simulink model "CryoDetHcd"  (R2016b)
settings: Solver=ode45  StartTime=0.0  StopTime=1e-3  RelTol=1e-3
PreLoadFcn:
  | setup_hcd
values from neighbouring files (symbols this model uses):
  A = sqrt(0.5*erfc(x))    [setup_hcd.m]
  etaRomData = zeros(1,128)    [setup_hcd.m]
  Fadc = 614e6    (= 614000000)    [setup_hcd.m]
  freqRomData = zeros(1,128)    [setup_hcd.m]
  freqRomData1 = zeros(1,128)    [setup_hcd.m]
  freqRomData2 = zeros(1,128)    [setup_hcd.m]
  freqRomData3 = zeros(1,128)    [setup_hcd.m]
undefined symbols (not defined in the file or in its folder): AXI4, B, C, D, j, Lite
libraries: xbsIndex_r4 x2151, CryoDetLibCMB x28, hdlsllib x8, dspsigops x2, simulink x1
(part 9 of 17)

== system CryoDetHcd/DspCore/DSP/channel_processor/channel_processor_x4/freqWord_debug/alpha_filter ==
  In1 : Inport
  alpha : Inport  Port=2
  ch : Inport  Port=3
  (D-A)*B + C : xbsIndex_r4/DSP48 Macro 3.0   dsptype=Target XtremeDSP Slice: DSP48E2  instruction_list=(D-A)*B+C  AvailableInstructions=|  show_filtered=on  pipeline_options=Expert  dspimage=?  tier_1=off  tier_2=off  tier_3=off  tier_4=off  tier_5=off  tier_6=off  dreg_1=off  dreg_2=off  dreg_3=on  areg_1=off  areg_2=off  areg_3=on  areg_4=on  breg_1=off  breg_2=off  breg_3=on  breg_4=on  mreg_5=on  concatreg_3=off  concatreg_4=off  concatreg_5=off  creg_1=off  creg_2=off  creg_3=on  creg_4=on  creg_5=on  preg_6=on  cinreg_1=off  cinreg_2=off  cinreg_3=off  cinreg_4=off  cinreg_5=off  opreg_1=off  opreg_2=off  opreg_3=off  opreg_4=off  opreg_5=off  output_properties=Full_Precision  p_width=48  p_binarywidth=0  has_acout=off  has_bcout=off  has_pcout=off  has_carryout=off  has_carrycascout=off  has_ce=off  has_d_ce=off  has_a_ce=off  has_b_ce=off  has_concat_ce=off  has_c_ce=off  has_m_ce=off  has_p_ce=off  has_sel_ce=off  has_sclr=off  has_d_sclr=off  has_a_sclr=off  has_b_sclr=off  has_concat_sclr=off  has_c_sclr=off  has_m_sclr=off  has_p_sclr=off  has_sel_sclr=off  use_dsp48=on  simulation_type=fast_sim  simulation_model=sysgen:xbip_dsp48_macro_v3_0  gui_behaviour=Sysgen  instruction1='#'  ip_name=DSP48 Macro  ip_version=3.0  dsptool_ready=true  ipcore_usecache=true  ipcore_useipmodelcache=true  wrapper_available=true  port_translation_map={ 'ce' => 'en', 'sclr' => 'rst'}  ipcore_latency_function='has_combinational'  structural_sim=false  ipcore_verbose=false  ipcore_port_config={ 'carryin' => { 'arith' => 'ufix', 'binpt' => 0.00000000000, 'width' => 1.00000000000}, 'carrycascin' => { 'arith' => 'ufix', 'binpt' => 0.00000000000, 'width' => 1.00000000000}, 'carrycascout' => { 'arith' => 'ufix', 'binpt' => 0.00000000000, 'width' => 1.00000000000}, 'carryout' => { 'arith' => 'ufix', 'binpt' => 0.00000000000, 'width' => 1.00000000000}}  ipcore_xco_need_fpga_part=true  block_type=xbip_dsp48_macro_v3_0
      | (D-A)*B+C
      | (D-A)*B+C+C
      | (D-A)*B+C+C+CARRYIN
      | (D-A)*B+C+CARRYIN
      | (D-A)*B+C+P
      | (D-A)*B+C+P+CARRYIN
      | (D-A)*B+C+P>>17
      | (D-A)*B+C+P>>17+CARRYIN
      | (D-A)*B+C+PCIN
      | (D-A)*B+C+PCIN+CARRYIN
      | (D-A)*B+C+PCIN>>17
      | (D-A)*B+C+PCIN>>17+CARRYIN
      | (D-A)*B+C-C
      | (D-A)*B+C-P
      | (D-A)*B+C-P>>17
      | (D-A)*B+C-PCIN
      | (D-A)*B+C-PCIN>>17
      | (D-A)*B+CARRYIN
      | -((D-A)*B+C)
      | -((D-A)*B+C+CARRYIN)
      | -((D-A)*B+CARRYIN)
      | -(C+(D-A)*B+CARRYIN)
      | -(P+(D-A)*B+CARRYIN)
      | -C+(D-A)*B+C
      | -P+(D-A)*B+C
      | -P>>17+(D-A)*B+C
      | -PCIN+(D-A)*B+C
      | -PCIN>>17+(D-A)*B+C
      | C+(D-A)*B+C
      | C+(D-A)*B+C+CARRYIN
      | C+(D-A)*B+CARRYIN
      | C+C+(D-A)*B+CARRYIN
      | C+P+(D-A)*B+CARRYIN
      | C+P>>17+(D-A)*B+CARRYIN
      | C+PCIN+(D-A)*B+CARRYIN
      | C+PCIN>>17+(D-A)*B+CARRYIN
      | C-((D-A)*B+C)
      | C-((D-A)*B+C+CARRYIN)
      | C-((D-A)*B+CARRYIN)
      | C-(C+(D-A)*B+CARRYIN)
      | C-(P+(D-A)*B+CARRYIN)
      | P+(D-A)*B+C
      | P+(D-A)*B+C+CARRYIN
      | P+(D-A)*B+CARRYIN
      | P+C+(D-A)*B+CARRYIN
      | P+P+(D-A)*B+CARRYIN
      | P+P>>17+(D-A)*B+CARRYIN
      | P+PCIN+(D-A)*B+CARRYIN
      | P+PCIN>>17+(D-A)*B+CARRYIN
      | P-((D-A)*B+C)
      | P-((D-A)*B+C+CARRYIN)
      | P-((D-A)*B+CARRYIN)
      | P-(C+(D-A)*B+CARRYIN)
      | P-(P+(D-A)*B+CARRYIN)
      | P>>17+(D-A)*B+C
      | P>>17+(D-A)*B+C+CARRYIN
      | P>>17+(D-A)*B+CARRYIN
      | P>>17+C+(D-A)*B+CARRYIN
      | P>>17+P+(D-A)*B+CARRYIN
      | P>>17-((D-A)*B+C)
      | P>>17-((D-A)*B+C+CARRYIN)
      | P>>17-((D-A)*B+CARRYIN)
      | P>>17-(C+(D-A)*B+CARRYIN)
      | P>>17-(P+(D-A)*B+CARRYIN)
      | PCIN+(D-A)*B+C
      | PCIN+(D-A)*B+C+CARRYIN
      | PCIN+(D-A)*B+CARRYIN
      | PCIN+C+(D-A)*B+CARRYIN
      | PCIN+P+(D-A)*B+CARRYIN
      | PCIN-((D-A)*B+C)
      | PCIN-((D-A)*B+C+CARRYIN)
      | PCIN-((D-A)*B+CARRYIN)
      | PCIN-(C+(D-A)*B+CARRYIN)
      | PCIN-(P+(D-A)*B+CARRYIN)
      | PCIN>>17+(D-A)*B+C
      | PCIN>>17+(D-A)*B+C+CARRYIN
      | PCIN>>17+(D-A)*B+CARRYIN
      | PCIN>>17+C+(D-A)*B+CARRYIN
      | PCIN>>17+P+(D-A)*B+CARRYIN
      | PCIN>>17-((D-A)*B+C)
      | PCIN>>17-((D-A)*B+C+CARRYIN)
      | PCIN>>17-((D-A)*B+CARRYIN)
      | PCIN>>17-(C+(D-A)*B+CARRYIN)
      | PCIN>>17-(P+(D-A)*B+CARRYIN)
      | RNDMACC((D-A)*B+C+P)
      | RNDSIMPLE((D-A)*B+C)
      | RNDSIMPLE((D-A)*B+C+CARRYIN)
      | RNDSIMPLE((D-A)*B+CARRYIN)
      | RNDSIMPLE(C+(D-A)*B+CARRYIN)
      | RNDSIMPLE(P+(D-A)*B+CARRYIN)
      | RNDSIMPLE(P>>17+(D-A)*B+CARRYIN)
      | RNDSIMPLE(PCIN+(D-A)*B+CARRYIN)
      | RNDSIMPLE(PCIN>>17+(D-A)*B+CARRYIN)
      settings: infoedit=<html>Valid operands: CONCAT, P, C, PCIN, P>>17, PCIN>>17, CARRYIN, CARRYCASCIN, ACIN, A, BCIN,B<br><br>Valid operators: +, -, *, ()<br><br>Valid functions: RNDSIMPLE, RNDSYM<br><br>Instructions are case insensitive and tolerate spaces.</html>
  Convert : xbsIndex_r4/Convert  gui_display_data_type=Fixed-point  arith_type=Unsigned  n_bits=24  bin_pt=0  float_type=Single  exp_bits=8  fraction_bits=24  quantization=Truncate  overflow=Wrap  en=off  latency=0  pipeline=off  dbl_ovrd=off  block_type=convert
  Convert1 : xbsIndex_r4/Convert  gui_display_data_type=Fixed-point  arith_type="Signed  (2's comp)"  n_bits=25  bin_pt=0  float_type=Single  exp_bits=8  fraction_bits=24  quantization=Truncate  overflow=Wrap  en=off  latency=0  pipeline=off  dbl_ovrd=off  block_type=convert
  Convert2 : xbsIndex_r4/Convert  gui_display_data_type=Fixed-point  arith_type="Signed  (2's comp)"  n_bits=18  bin_pt=15  float_type=Single  exp_bits=8  fraction_bits=24  quantization=Truncate  overflow=Wrap  en=off  latency=0  pipeline=off  dbl_ovrd=off  block_type=convert
  Convert3 : xbsIndex_r4/Convert  gui_display_data_type=Fixed-point  arith_type="Signed  (2's comp)"  n_bits=25  bin_pt=0  float_type=Single  exp_bits=8  fraction_bits=24  quantization=Truncate  overflow=Wrap  en=off  latency=0  pipeline=off  dbl_ovrd=off  block_type=convert
  Delay : xbsIndex_r4/Delay  rst=off  infoeditControl=Selection of Reset will increase slice count due to use of real FFs and instead of SRLs  en=off  latency=4  reg_retiming=off  dbl_ovrd=off  block_type=delay
  Delay1 : xbsIndex_r4/Delay  rst=off  infoeditControl=Selection of Reset will increase slice count due to use of real FFs and instead of SRLs  en=off  latency=4  reg_retiming=off  dbl_ovrd=off  block_type=delay
  Register : xbsIndex_r4/Register  init=0  rst=off  en=off  dbl_ovrd=off  block_type=register
  Out1 : Outport
  ch_o : Outport  Port=2
  wires:
  Register/1 -> Convert3/1
  In1/1 -> Register/1
  Delay/1 -> Convert1/1, (D-A)*B + C/4
  (D-A)*B + C/1 -> Convert/1, Delay/1
  Convert1/1 -> (D-A)*B + C/2
  Convert/1 -> Out1/1
  Convert2/1 -> (D-A)*B + C/3
  Convert3/1 -> (D-A)*B + C/1
  ch/1 -> Delay1/1
  Delay1/1 -> ch_o/1
  alpha/1 -> Convert2/1

== system CryoDetHcd/DspCore/DSP/channel_processor/channel_processor_x4/freqWord_debug/alpha_filter1 ==
  In1 : Inport
  alpha : Inport  Port=2
  ch : Inport  Port=3
  (D-A)*B + C : xbsIndex_r4/DSP48 Macro 3.0   dsptype=Target XtremeDSP Slice: DSP48E2  instruction_list=(D-A)*B+C  AvailableInstructions=|  show_filtered=on  pipeline_options=Expert  dspimage=?  tier_1=off  tier_2=off  tier_3=off  tier_4=off  tier_5=off  tier_6=off  dreg_1=off  dreg_2=off  dreg_3=on  areg_1=off  areg_2=off  areg_3=on  areg_4=on  breg_1=off  breg_2=off  breg_3=on  breg_4=on  mreg_5=on  concatreg_3=off  concatreg_4=off  concatreg_5=off  creg_1=off  creg_2=off  creg_3=on  creg_4=on  creg_5=on  preg_6=on  cinreg_1=off  cinreg_2=off  cinreg_3=off  cinreg_4=off  cinreg_5=off  opreg_1=off  opreg_2=off  opreg_3=off  opreg_4=off  opreg_5=off  output_properties=Full_Precision  p_width=48  p_binarywidth=0  has_acout=off  has_bcout=off  has_pcout=off  has_carryout=off  has_carrycascout=off  has_ce=off  has_d_ce=off  has_a_ce=off  has_b_ce=off  has_concat_ce=off  has_c_ce=off  has_m_ce=off  has_p_ce=off  has_sel_ce=off  has_sclr=off  has_d_sclr=off  has_a_sclr=off  has_b_sclr=off  has_concat_sclr=off  has_c_sclr=off  has_m_sclr=off  has_p_sclr=off  has_sel_sclr=off  use_dsp48=on  simulation_type=fast_sim  simulation_model=sysgen:xbip_dsp48_macro_v3_0  gui_behaviour=Sysgen  instruction1='#'  ip_name=DSP48 Macro  ip_version=3.0  dsptool_ready=true  ipcore_usecache=true  ipcore_useipmodelcache=true  wrapper_available=true  port_translation_map={ 'ce' => 'en', 'sclr' => 'rst'}  ipcore_latency_function='has_combinational'  structural_sim=false  ipcore_verbose=false  ipcore_port_config={ 'carryin' => { 'arith' => 'ufix', 'binpt' => 0.00000000000, 'width' => 1.00000000000}, 'carrycascin' => { 'arith' => 'ufix', 'binpt' => 0.00000000000, 'width' => 1.00000000000}, 'carrycascout' => { 'arith' => 'ufix', 'binpt' => 0.00000000000, 'width' => 1.00000000000}, 'carryout' => { 'arith' => 'ufix', 'binpt' => 0.00000000000, 'width' => 1.00000000000}}  ipcore_xco_need_fpga_part=true  block_type=xbip_dsp48_macro_v3_0
      | (D-A)*B+C
      | (D-A)*B+C+C
      | (D-A)*B+C+C+CARRYIN
      | (D-A)*B+C+CARRYIN
      | (D-A)*B+C+P
      | (D-A)*B+C+P+CARRYIN
      | (D-A)*B+C+P>>17
      | (D-A)*B+C+P>>17+CARRYIN
      | (D-A)*B+C+PCIN
      | (D-A)*B+C+PCIN+CARRYIN
      | (D-A)*B+C+PCIN>>17
      | (D-A)*B+C+PCIN>>17+CARRYIN
      | (D-A)*B+C-C
      | (D-A)*B+C-P
      | (D-A)*B+C-P>>17
      | (D-A)*B+C-PCIN
      | (D-A)*B+C-PCIN>>17
      | (D-A)*B+CARRYIN
      | -((D-A)*B+C)
      | -((D-A)*B+C+CARRYIN)
      | -((D-A)*B+CARRYIN)
      | -(C+(D-A)*B+CARRYIN)
      | -(P+(D-A)*B+CARRYIN)
      | -C+(D-A)*B+C
      | -P+(D-A)*B+C
      | -P>>17+(D-A)*B+C
      | -PCIN+(D-A)*B+C
      | -PCIN>>17+(D-A)*B+C
      | C+(D-A)*B+C
      | C+(D-A)*B+C+CARRYIN
      | C+(D-A)*B+CARRYIN
      | C+C+(D-A)*B+CARRYIN
      | C+P+(D-A)*B+CARRYIN
      | C+P>>17+(D-A)*B+CARRYIN
      | C+PCIN+(D-A)*B+CARRYIN
      | C+PCIN>>17+(D-A)*B+CARRYIN
      | C-((D-A)*B+C)
      | C-((D-A)*B+C+CARRYIN)
      | C-((D-A)*B+CARRYIN)
      | C-(C+(D-A)*B+CARRYIN)
      | C-(P+(D-A)*B+CARRYIN)
      | P+(D-A)*B+C
      | P+(D-A)*B+C+CARRYIN
      | P+(D-A)*B+CARRYIN
      | P+C+(D-A)*B+CARRYIN
      | P+P+(D-A)*B+CARRYIN
      | P+P>>17+(D-A)*B+CARRYIN
      | P+PCIN+(D-A)*B+CARRYIN
      | P+PCIN>>17+(D-A)*B+CARRYIN
      | P-((D-A)*B+C)
      | P-((D-A)*B+C+CARRYIN)
      | P-((D-A)*B+CARRYIN)
      | P-(C+(D-A)*B+CARRYIN)
      | P-(P+(D-A)*B+CARRYIN)
      | P>>17+(D-A)*B+C
      | P>>17+(D-A)*B+C+CARRYIN
      | P>>17+(D-A)*B+CARRYIN
      | P>>17+C+(D-A)*B+CARRYIN
      | P>>17+P+(D-A)*B+CARRYIN
      | P>>17-((D-A)*B+C)
      | P>>17-((D-A)*B+C+CARRYIN)
      | P>>17-((D-A)*B+CARRYIN)
      | P>>17-(C+(D-A)*B+CARRYIN)
      | P>>17-(P+(D-A)*B+CARRYIN)
      | PCIN+(D-A)*B+C
      | PCIN+(D-A)*B+C+CARRYIN
      | PCIN+(D-A)*B+CARRYIN
      | PCIN+C+(D-A)*B+CARRYIN
      | PCIN+P+(D-A)*B+CARRYIN
      | PCIN-((D-A)*B+C)
      | PCIN-((D-A)*B+C+CARRYIN)
      | PCIN-((D-A)*B+CARRYIN)
      | PCIN-(C+(D-A)*B+CARRYIN)
      | PCIN-(P+(D-A)*B+CARRYIN)
      | PCIN>>17+(D-A)*B+C
      | PCIN>>17+(D-A)*B+C+CARRYIN
      | PCIN>>17+(D-A)*B+CARRYIN
      | PCIN>>17+C+(D-A)*B+CARRYIN
      | PCIN>>17+P+(D-A)*B+CARRYIN
      | PCIN>>17-((D-A)*B+C)
      | PCIN>>17-((D-A)*B+C+CARRYIN)
      | PCIN>>17-((D-A)*B+CARRYIN)
      | PCIN>>17-(C+(D-A)*B+CARRYIN)
      | PCIN>>17-(P+(D-A)*B+CARRYIN)
      | RNDMACC((D-A)*B+C+P)
      | RNDSIMPLE((D-A)*B+C)
      | RNDSIMPLE((D-A)*B+C+CARRYIN)
      | RNDSIMPLE((D-A)*B+CARRYIN)
      | RNDSIMPLE(C+(D-A)*B+CARRYIN)
      | RNDSIMPLE(P+(D-A)*B+CARRYIN)
      | RNDSIMPLE(P>>17+(D-A)*B+CARRYIN)
      | RNDSIMPLE(PCIN+(D-A)*B+CARRYIN)
      | RNDSIMPLE(PCIN>>17+(D-A)*B+CARRYIN)
      settings: infoedit=<html>Valid operands: CONCAT, P, C, PCIN, P>>17, PCIN>>17, CARRYIN, CARRYCASCIN, ACIN, A, BCIN,B<br><br>Valid operators: +, -, *, ()<br><br>Valid functions: RNDSIMPLE, RNDSYM<br><br>Instructions are case insensitive and tolerate spaces.</html>
  Convert : xbsIndex_r4/Convert  gui_display_data_type=Fixed-point  arith_type=Unsigned  n_bits=24  bin_pt=0  float_type=Single  exp_bits=8  fraction_bits=24  quantization=Truncate  overflow=Wrap  en=off  latency=0  pipeline=off  dbl_ovrd=off  block_type=convert
  Convert1 : xbsIndex_r4/Convert  gui_display_data_type=Fixed-point  arith_type="Signed  (2's comp)"  n_bits=25  bin_pt=0  float_type=Single  exp_bits=8  fraction_bits=24  quantization=Truncate  overflow=Wrap  en=off  latency=0  pipeline=off  dbl_ovrd=off  block_type=convert
  Convert2 : xbsIndex_r4/Convert  gui_display_data_type=Fixed-point  arith_type="Signed  (2's comp)"  n_bits=18  bin_pt=15  float_type=Single  exp_bits=8  fraction_bits=24  quantization=Truncate  overflow=Wrap  en=off  latency=0  pipeline=off  dbl_ovrd=off  block_type=convert
  Convert3 : xbsIndex_r4/Convert  gui_display_data_type=Fixed-point  arith_type="Signed  (2's comp)"  n_bits=25  bin_pt=0  float_type=Single  exp_bits=8  fraction_bits=24  quantization=Truncate  overflow=Wrap  en=off  latency=0  pipeline=off  dbl_ovrd=off  block_type=convert
  Delay : xbsIndex_r4/Delay  rst=off  infoeditControl=Selection of Reset will increase slice count due to use of real FFs and instead of SRLs  en=off  latency=4  reg_retiming=off  dbl_ovrd=off  block_type=delay
  Delay1 : xbsIndex_r4/Delay  rst=off  infoeditControl=Selection of Reset will increase slice count due to use of real FFs and instead of SRLs  en=off  latency=4  reg_retiming=off  dbl_ovrd=off  block_type=delay
  Register : xbsIndex_r4/Register  init=0  rst=off  en=off  dbl_ovrd=off  block_type=register
  Out1 : Outport
  ch_o : Outport  Port=2
  wires:
  alpha/1 -> Convert2/1
  Delay1/1 -> ch_o/1
  ch/1 -> Delay1/1
  Convert3/1 -> (D-A)*B + C/1
  Convert2/1 -> (D-A)*B + C/3
  Convert/1 -> Out1/1
  Convert1/1 -> (D-A)*B + C/2
  (D-A)*B + C/1 -> Delay/1, Convert/1
  Delay/1 -> (D-A)*B + C/4, Convert1/1
  In1/1 -> Register/1
  Register/1 -> Convert3/1

== system CryoDetHcd/DspCore/DSP/channel_processor/channel_processor_x4/freqWord_debug/alpha_filter2 ==
  In1 : Inport
  alpha : Inport  Port=2
  ch : Inport  Port=3
  (D-A)*B + C : xbsIndex_r4/DSP48 Macro 3.0   dsptype=Target XtremeDSP Slice: DSP48E2  instruction_list=(D-A)*B+C  AvailableInstructions=|  show_filtered=on  pipeline_options=Expert  dspimage=?  tier_1=off  tier_2=off  tier_3=off  tier_4=off  tier_5=off  tier_6=off  dreg_1=off  dreg_2=off  dreg_3=on  areg_1=off  areg_2=off  areg_3=on  areg_4=on  breg_1=off  breg_2=off  breg_3=on  breg_4=on  mreg_5=on  concatreg_3=off  concatreg_4=off  concatreg_5=off  creg_1=off  creg_2=off  creg_3=on  creg_4=on  creg_5=on  preg_6=on  cinreg_1=off  cinreg_2=off  cinreg_3=off  cinreg_4=off  cinreg_5=off  opreg_1=off  opreg_2=off  opreg_3=off  opreg_4=off  opreg_5=off  output_properties=Full_Precision  p_width=48  p_binarywidth=0  has_acout=off  has_bcout=off  has_pcout=off  has_carryout=off  has_carrycascout=off  has_ce=off  has_d_ce=off  has_a_ce=off  has_b_ce=off  has_concat_ce=off  has_c_ce=off  has_m_ce=off  has_p_ce=off  has_sel_ce=off  has_sclr=off  has_d_sclr=off  has_a_sclr=off  has_b_sclr=off  has_concat_sclr=off  has_c_sclr=off  has_m_sclr=off  has_p_sclr=off  has_sel_sclr=off  use_dsp48=on  simulation_type=fast_sim  simulation_model=sysgen:xbip_dsp48_macro_v3_0  gui_behaviour=Sysgen  instruction1='#'  ip_name=DSP48 Macro  ip_version=3.0  dsptool_ready=true  ipcore_usecache=true  ipcore_useipmodelcache=true  wrapper_available=true  port_translation_map={ 'ce' => 'en', 'sclr' => 'rst'}  ipcore_latency_function='has_combinational'  structural_sim=false  ipcore_verbose=false  ipcore_port_config={ 'carryin' => { 'arith' => 'ufix', 'binpt' => 0.00000000000, 'width' => 1.00000000000}, 'carrycascin' => { 'arith' => 'ufix', 'binpt' => 0.00000000000, 'width' => 1.00000000000}, 'carrycascout' => { 'arith' => 'ufix', 'binpt' => 0.00000000000, 'width' => 1.00000000000}, 'carryout' => { 'arith' => 'ufix', 'binpt' => 0.00000000000, 'width' => 1.00000000000}}  ipcore_xco_need_fpga_part=true  block_type=xbip_dsp48_macro_v3_0
      | (D-A)*B+C
      | (D-A)*B+C+C
      | (D-A)*B+C+C+CARRYIN
      | (D-A)*B+C+CARRYIN
      | (D-A)*B+C+P
      | (D-A)*B+C+P+CARRYIN
      | (D-A)*B+C+P>>17
      | (D-A)*B+C+P>>17+CARRYIN
      | (D-A)*B+C+PCIN
      | (D-A)*B+C+PCIN+CARRYIN
      | (D-A)*B+C+PCIN>>17
      | (D-A)*B+C+PCIN>>17+CARRYIN
      | (D-A)*B+C-C
      | (D-A)*B+C-P
      | (D-A)*B+C-P>>17
      | (D-A)*B+C-PCIN
      | (D-A)*B+C-PCIN>>17
      | (D-A)*B+CARRYIN
      | -((D-A)*B+C)
      | -((D-A)*B+C+CARRYIN)
      | -((D-A)*B+CARRYIN)
      | -(C+(D-A)*B+CARRYIN)
      | -(P+(D-A)*B+CARRYIN)
      | -C+(D-A)*B+C
      | -P+(D-A)*B+C
      | -P>>17+(D-A)*B+C
      | -PCIN+(D-A)*B+C
      | -PCIN>>17+(D-A)*B+C
      | C+(D-A)*B+C
      | C+(D-A)*B+C+CARRYIN
      | C+(D-A)*B+CARRYIN
      | C+C+(D-A)*B+CARRYIN
      | C+P+(D-A)*B+CARRYIN
      | C+P>>17+(D-A)*B+CARRYIN
      | C+PCIN+(D-A)*B+CARRYIN
      | C+PCIN>>17+(D-A)*B+CARRYIN
      | C-((D-A)*B+C)
      | C-((D-A)*B+C+CARRYIN)
      | C-((D-A)*B+CARRYIN)
      | C-(C+(D-A)*B+CARRYIN)
      | C-(P+(D-A)*B+CARRYIN)
      | P+(D-A)*B+C
      | P+(D-A)*B+C+CARRYIN
      | P+(D-A)*B+CARRYIN
      | P+C+(D-A)*B+CARRYIN
      | P+P+(D-A)*B+CARRYIN
      | P+P>>17+(D-A)*B+CARRYIN
      | P+PCIN+(D-A)*B+CARRYIN
      | P+PCIN>>17+(D-A)*B+CARRYIN
      | P-((D-A)*B+C)
      | P-((D-A)*B+C+CARRYIN)
      | P-((D-A)*B+CARRYIN)
      | P-(C+(D-A)*B+CARRYIN)
      | P-(P+(D-A)*B+CARRYIN)
      | P>>17+(D-A)*B+C
      | P>>17+(D-A)*B+C+CARRYIN
      | P>>17+(D-A)*B+CARRYIN
      | P>>17+C+(D-A)*B+CARRYIN
      | P>>17+P+(D-A)*B+CARRYIN
      | P>>17-((D-A)*B+C)
      | P>>17-((D-A)*B+C+CARRYIN)
      | P>>17-((D-A)*B+CARRYIN)
      | P>>17-(C+(D-A)*B+CARRYIN)
      | P>>17-(P+(D-A)*B+CARRYIN)
      | PCIN+(D-A)*B+C
      | PCIN+(D-A)*B+C+CARRYIN
      | PCIN+(D-A)*B+CARRYIN
      | PCIN+C+(D-A)*B+CARRYIN
      | PCIN+P+(D-A)*B+CARRYIN
      | PCIN-((D-A)*B+C)
      | PCIN-((D-A)*B+C+CARRYIN)
      | PCIN-((D-A)*B+CARRYIN)
      | PCIN-(C+(D-A)*B+CARRYIN)
      | PCIN-(P+(D-A)*B+CARRYIN)
      | PCIN>>17+(D-A)*B+C
      | PCIN>>17+(D-A)*B+C+CARRYIN
      | PCIN>>17+(D-A)*B+CARRYIN
      | PCIN>>17+C+(D-A)*B+CARRYIN
      | PCIN>>17+P+(D-A)*B+CARRYIN
      | PCIN>>17-((D-A)*B+C)
      | PCIN>>17-((D-A)*B+C+CARRYIN)
      | PCIN>>17-((D-A)*B+CARRYIN)
      | PCIN>>17-(C+(D-A)*B+CARRYIN)
      | PCIN>>17-(P+(D-A)*B+CARRYIN)
      | RNDMACC((D-A)*B+C+P)
      | RNDSIMPLE((D-A)*B+C)
      | RNDSIMPLE((D-A)*B+C+CARRYIN)
      | RNDSIMPLE((D-A)*B+CARRYIN)
      | RNDSIMPLE(C+(D-A)*B+CARRYIN)
      | RNDSIMPLE(P+(D-A)*B+CARRYIN)
      | RNDSIMPLE(P>>17+(D-A)*B+CARRYIN)
      | RNDSIMPLE(PCIN+(D-A)*B+CARRYIN)
      | RNDSIMPLE(PCIN>>17+(D-A)*B+CARRYIN)
      settings: infoedit=<html>Valid operands: CONCAT, P, C, PCIN, P>>17, PCIN>>17, CARRYIN, CARRYCASCIN, ACIN, A, BCIN,B<br><br>Valid operators: +, -, *, ()<br><br>Valid functions: RNDSIMPLE, RNDSYM<br><br>Instructions are case insensitive and tolerate spaces.</html>
  Convert : xbsIndex_r4/Convert  gui_display_data_type=Fixed-point  arith_type=Unsigned  n_bits=24  bin_pt=0  float_type=Single  exp_bits=8  fraction_bits=24  quantization=Truncate  overflow=Wrap  en=off  latency=0  pipeline=off  dbl_ovrd=off  block_type=convert
  Convert1 : xbsIndex_r4/Convert  gui_display_data_type=Fixed-point  arith_type="Signed  (2's comp)"  n_bits=25  bin_pt=0  float_type=Single  exp_bits=8  fraction_bits=24  quantization=Truncate  overflow=Wrap  en=off  latency=0  pipeline=off  dbl_ovrd=off  block_type=convert
  Convert2 : xbsIndex_r4/Convert  gui_display_data_type=Fixed-point  arith_type="Signed  (2's comp)"  n_bits=18  bin_pt=15  float_type=Single  exp_bits=8  fraction_bits=24  quantization=Truncate  overflow=Wrap  en=off  latency=0  pipeline=off  dbl_ovrd=off  block_type=convert
  Convert3 : xbsIndex_r4/Convert  gui_display_data_type=Fixed-point  arith_type="Signed  (2's comp)"  n_bits=25  bin_pt=0  float_type=Single  exp_bits=8  fraction_bits=24  quantization=Truncate  overflow=Wrap  en=off  latency=0  pipeline=off  dbl_ovrd=off  block_type=convert
  Delay : xbsIndex_r4/Delay  rst=off  infoeditControl=Selection of Reset will increase slice count due to use of real FFs and instead of SRLs  en=off  latency=4  reg_retiming=off  dbl_ovrd=off  block_type=delay
  Delay1 : xbsIndex_r4/Delay  rst=off  infoeditControl=Selection of Reset will increase slice count due to use of real FFs and instead of SRLs  en=off  latency=4  reg_retiming=off  dbl_ovrd=off  block_type=delay
  Register : xbsIndex_r4/Register  init=0  rst=off  en=off  dbl_ovrd=off  block_type=register
  Out1 : Outport
  ch_o : Outport  Port=2
  wires:
  Register/1 -> Convert3/1
  In1/1 -> Register/1
  Delay/1 -> Convert1/1, (D-A)*B + C/4
  (D-A)*B + C/1 -> Convert/1, Delay/1
  Convert1/1 -> (D-A)*B + C/2
  Convert/1 -> Out1/1
  Convert2/1 -> (D-A)*B + C/3
  Convert3/1 -> (D-A)*B + C/1
  ch/1 -> Delay1/1
  Delay1/1 -> ch_o/1
  alpha/1 -> Convert2/1

== system CryoDetHcd/DspCore/DSP/channel_processor/channel_processor_x4/freqWord_debug/alpha_filter3 ==
  In1 : Inport
  alpha : Inport  Port=2
  ch : Inport  Port=3
  (D-A)*B + C : xbsIndex_r4/DSP48 Macro 3.0   dsptype=Target XtremeDSP Slice: DSP48E2  instruction_list=(D-A)*B+C  AvailableInstructions=|  show_filtered=on  pipeline_options=Expert  dspimage=?  tier_1=off  tier_2=off  tier_3=off  tier_4=off  tier_5=off  tier_6=off  dreg_1=off  dreg_2=off  dreg_3=on  areg_1=off  areg_2=off  areg_3=on  areg_4=on  breg_1=off  breg_2=off  breg_3=on  breg_4=on  mreg_5=on  concatreg_3=off  concatreg_4=off  concatreg_5=off  creg_1=off  creg_2=off  creg_3=on  creg_4=on  creg_5=on  preg_6=on  cinreg_1=off  cinreg_2=off  cinreg_3=off  cinreg_4=off  cinreg_5=off  opreg_1=off  opreg_2=off  opreg_3=off  opreg_4=off  opreg_5=off  output_properties=Full_Precision  p_width=48  p_binarywidth=0  has_acout=off  has_bcout=off  has_pcout=off  has_carryout=off  has_carrycascout=off  has_ce=off  has_d_ce=off  has_a_ce=off  has_b_ce=off  has_concat_ce=off  has_c_ce=off  has_m_ce=off  has_p_ce=off  has_sel_ce=off  has_sclr=off  has_d_sclr=off  has_a_sclr=off  has_b_sclr=off  has_concat_sclr=off  has_c_sclr=off  has_m_sclr=off  has_p_sclr=off  has_sel_sclr=off  use_dsp48=on  simulation_type=fast_sim  simulation_model=sysgen:xbip_dsp48_macro_v3_0  gui_behaviour=Sysgen  instruction1='#'  ip_name=DSP48 Macro  ip_version=3.0  dsptool_ready=true  ipcore_usecache=true  ipcore_useipmodelcache=true  wrapper_available=true  port_translation_map={ 'ce' => 'en', 'sclr' => 'rst'}  ipcore_latency_function='has_combinational'  structural_sim=false  ipcore_verbose=false  ipcore_port_config={ 'carryin' => { 'arith' => 'ufix', 'binpt' => 0.00000000000, 'width' => 1.00000000000}, 'carrycascin' => { 'arith' => 'ufix', 'binpt' => 0.00000000000, 'width' => 1.00000000000}, 'carrycascout' => { 'arith' => 'ufix', 'binpt' => 0.00000000000, 'width' => 1.00000000000}, 'carryout' => { 'arith' => 'ufix', 'binpt' => 0.00000000000, 'width' => 1.00000000000}}  ipcore_xco_need_fpga_part=true  block_type=xbip_dsp48_macro_v3_0
      | (D-A)*B+C
      | (D-A)*B+C+C
      | (D-A)*B+C+C+CARRYIN
      | (D-A)*B+C+CARRYIN
      | (D-A)*B+C+P
      | (D-A)*B+C+P+CARRYIN
      | (D-A)*B+C+P>>17
      | (D-A)*B+C+P>>17+CARRYIN
      | (D-A)*B+C+PCIN
      | (D-A)*B+C+PCIN+CARRYIN
      | (D-A)*B+C+PCIN>>17
      | (D-A)*B+C+PCIN>>17+CARRYIN
      | (D-A)*B+C-C
      | (D-A)*B+C-P
      | (D-A)*B+C-P>>17
      | (D-A)*B+C-PCIN
      | (D-A)*B+C-PCIN>>17
      | (D-A)*B+CARRYIN
      | -((D-A)*B+C)
      | -((D-A)*B+C+CARRYIN)
      | -((D-A)*B+CARRYIN)
      | -(C+(D-A)*B+CARRYIN)
      | -(P+(D-A)*B+CARRYIN)
      | -C+(D-A)*B+C
      | -P+(D-A)*B+C
      | -P>>17+(D-A)*B+C
      | -PCIN+(D-A)*B+C
      | -PCIN>>17+(D-A)*B+C
      | C+(D-A)*B+C
      | C+(D-A)*B+C+CARRYIN
      | C+(D-A)*B+CARRYIN
      | C+C+(D-A)*B+CARRYIN
      | C+P+(D-A)*B+CARRYIN
      | C+P>>17+(D-A)*B+CARRYIN
      | C+PCIN+(D-A)*B+CARRYIN
      | C+PCIN>>17+(D-A)*B+CARRYIN
      | C-((D-A)*B+C)
      | C-((D-A)*B+C+CARRYIN)
      | C-((D-A)*B+CARRYIN)
      | C-(C+(D-A)*B+CARRYIN)
      | C-(P+(D-A)*B+CARRYIN)
      | P+(D-A)*B+C
      | P+(D-A)*B+C+CARRYIN
      | P+(D-A)*B+CARRYIN
      | P+C+(D-A)*B+CARRYIN
      | P+P+(D-A)*B+CARRYIN
      | P+P>>17+(D-A)*B+CARRYIN
      | P+PCIN+(D-A)*B+CARRYIN
      | P+PCIN>>17+(D-A)*B+CARRYIN
      | P-((D-A)*B+C)
      | P-((D-A)*B+C+CARRYIN)
      | P-((D-A)*B+CARRYIN)
      | P-(C+(D-A)*B+CARRYIN)
      | P-(P+(D-A)*B+CARRYIN)
      | P>>17+(D-A)*B+C
      | P>>17+(D-A)*B+C+CARRYIN
      | P>>17+(D-A)*B+CARRYIN
      | P>>17+C+(D-A)*B+CARRYIN
      | P>>17+P+(D-A)*B+CARRYIN
      | P>>17-((D-A)*B+C)
      | P>>17-((D-A)*B+C+CARRYIN)
      | P>>17-((D-A)*B+CARRYIN)
      | P>>17-(C+(D-A)*B+CARRYIN)
      | P>>17-(P+(D-A)*B+CARRYIN)
      | PCIN+(D-A)*B+C
      | PCIN+(D-A)*B+C+CARRYIN
      | PCIN+(D-A)*B+CARRYIN
      | PCIN+C+(D-A)*B+CARRYIN
      | PCIN+P+(D-A)*B+CARRYIN
      | PCIN-((D-A)*B+C)
      | PCIN-((D-A)*B+C+CARRYIN)
      | PCIN-((D-A)*B+CARRYIN)
      | PCIN-(C+(D-A)*B+CARRYIN)
      | PCIN-(P+(D-A)*B+CARRYIN)
      | PCIN>>17+(D-A)*B+C
      | PCIN>>17+(D-A)*B+C+CARRYIN
      | PCIN>>17+(D-A)*B+CARRYIN
      | PCIN>>17+C+(D-A)*B+CARRYIN
      | PCIN>>17+P+(D-A)*B+CARRYIN
      | PCIN>>17-((D-A)*B+C)
      | PCIN>>17-((D-A)*B+C+CARRYIN)
      | PCIN>>17-((D-A)*B+CARRYIN)
      | PCIN>>17-(C+(D-A)*B+CARRYIN)
      | PCIN>>17-(P+(D-A)*B+CARRYIN)
      | RNDMACC((D-A)*B+C+P)
      | RNDSIMPLE((D-A)*B+C)
      | RNDSIMPLE((D-A)*B+C+CARRYIN)
      | RNDSIMPLE((D-A)*B+CARRYIN)
      | RNDSIMPLE(C+(D-A)*B+CARRYIN)
      | RNDSIMPLE(P+(D-A)*B+CARRYIN)
      | RNDSIMPLE(P>>17+(D-A)*B+CARRYIN)
      | RNDSIMPLE(PCIN+(D-A)*B+CARRYIN)
      | RNDSIMPLE(PCIN>>17+(D-A)*B+CARRYIN)
      settings: infoedit=<html>Valid operands: CONCAT, P, C, PCIN, P>>17, PCIN>>17, CARRYIN, CARRYCASCIN, ACIN, A, BCIN,B<br><br>Valid operators: +, -, *, ()<br><br>Valid functions: RNDSIMPLE, RNDSYM<br><br>Instructions are case insensitive and tolerate spaces.</html>
  Convert : xbsIndex_r4/Convert  gui_display_data_type=Fixed-point  arith_type=Unsigned  n_bits=24  bin_pt=0  float_type=Single  exp_bits=8  fraction_bits=24  quantization=Truncate  overflow=Wrap  en=off  latency=0  pipeline=off  dbl_ovrd=off  block_type=convert
  Convert1 : xbsIndex_r4/Convert  gui_display_data_type=Fixed-point  arith_type="Signed  (2's comp)"  n_bits=25  bin_pt=0  float_type=Single  exp_bits=8  fraction_bits=24  quantization=Truncate  overflow=Wrap  en=off  latency=0  pipeline=off  dbl_ovrd=off  block_type=convert
  Convert2 : xbsIndex_r4/Convert  gui_display_data_type=Fixed-point  arith_type="Signed  (2's comp)"  n_bits=18  bin_pt=15  float_type=Single  exp_bits=8  fraction_bits=24  quantization=Truncate  overflow=Wrap  en=off  latency=0  pipeline=off  dbl_ovrd=off  block_type=convert
  Convert3 : xbsIndex_r4/Convert  gui_display_data_type=Fixed-point  arith_type="Signed  (2's comp)"  n_bits=25  bin_pt=0  float_type=Single  exp_bits=8  fraction_bits=24  quantization=Truncate  overflow=Wrap  en=off  latency=0  pipeline=off  dbl_ovrd=off  block_type=convert
  Delay : xbsIndex_r4/Delay  rst=off  infoeditControl=Selection of Reset will increase slice count due to use of real FFs and instead of SRLs  en=off  latency=4  reg_retiming=off  dbl_ovrd=off  block_type=delay
  Delay1 : xbsIndex_r4/Delay  rst=off  infoeditControl=Selection of Reset will increase slice count due to use of real FFs and instead of SRLs  en=off  latency=4  reg_retiming=off  dbl_ovrd=off  block_type=delay
  Register : xbsIndex_r4/Register  init=0  rst=off  en=off  dbl_ovrd=off  block_type=register
  Out1 : Outport
  ch_o : Outport  Port=2
  wires:
  alpha/1 -> Convert2/1
  Delay1/1 -> ch_o/1
  ch/1 -> Delay1/1
  Convert3/1 -> (D-A)*B + C/1
  Convert2/1 -> (D-A)*B + C/3
  Convert/1 -> Out1/1
  Convert1/1 -> (D-A)*B + C/2
  (D-A)*B + C/1 -> Delay/1, Convert/1
  Delay/1 -> (D-A)*B + C/4, Convert1/1
  In1/1 -> Register/1
  Register/1 -> Convert3/1

== system CryoDetHcd/DspCore/DSP/channel_processor/channel_processor_x4/128_channel_processor1/DDS Mixer taylor series corrected/DDS 8ch taylor series corrected ==
  note: Taylor series corrected - use 0.5 BRAM (18 bit storage, 2^10 points), 3DSP
  note: Phase Accumulator
      | (8 Channels)
  note: 8 Channel DDS
      | Given its channel ID, takes instantaneous frequency for this channel of each band and generates phase and I&Q
      | interleaved over 8 bands
      | Frequency RAM is updated asynchronously to operation
  note: don't worry about matching latency here, will do downstream
  valid : Inport
  rst : Inport  Port=2
  freqWord : Inport  Port=3
  index : Inport  Port=4
  ch : Inport  Port=5
  BitBasher : xbsIndex_r4/BitBasher  bitexpr=tmux = {in[6:4]}  display_expr=off  sr_1=tmux  arith_type1=Unsigned  bin_pt1=0  sr_2=subband  arith_type2=Unsigned  bin_pt2=0  sr_3=3  arith_type3=Unsigned  bin_pt3=0  sr_4=4  arith_type4=Unsigned  bin_pt4=0  dbl_ovrd=off  block_type=bitbasher
  BitBasher1 : xbsIndex_r4/BitBasher  bitexpr=|  display_expr=off  sr_1=ch  arith_type1=Unsigned  bin_pt1=0  sr_2=amp  arith_type2=Unsigned  bin_pt2=0  sr_3=3  arith_type3=Unsigned  bin_pt3=0  sr_4=4  arith_type4=Unsigned  bin_pt4=0  dbl_ovrd=off  block_type=bitbasher
      | ch = {in[6:4]}
      | amp = {in[3:0]}
  BitBasher2 : xbsIndex_r4/BitBasher  bitexpr=|  display_expr=off  sr_1=freq  arith_type1=Unsigned  bin_pt1=24  sr_2=amp  arith_type2=Unsigned  bin_pt2=0  sr_3=3  arith_type3=Unsigned  bin_pt3=0  sr_4=4  arith_type4=Unsigned  bin_pt4=0  dbl_ovrd=off  block_type=bitbasher
      | freq = {in[23:0]}
      | amp = {in[27:24]}
  BitBasher3 : xbsIndex_r4/BitBasher  bitexpr=out = {ch, amp}  display_expr=off  sr_1=out  arith_type1=Unsigned  bin_pt1=0  sr_2=amp  arith_type2=Unsigned  bin_pt2=0  sr_3=3  arith_type3=Unsigned  bin_pt3=0  sr_4=4  arith_type4=Unsigned  bin_pt4=0  dbl_ovrd=off  block_type=bitbasher
  BitBasher4 : xbsIndex_r4/BitBasher  bitexpr=|  display_expr=off  sr_1=ch  arith_type1=Unsigned  bin_pt1=0  sr_2=amp  arith_type2=Unsigned  bin_pt2=0  sr_3=3  arith_type3=Unsigned  bin_pt3=0  sr_4=4  arith_type4=Unsigned  bin_pt4=0  dbl_ovrd=off  block_type=bitbasher
      | ch = {in[6:4]}
      | amp = {in[3:0]}
  BitBasher5 : xbsIndex_r4/BitBasher  bitexpr=phase = {in[23:8]}  display_expr=off  sr_1=phase  arith_type1="Signed  (2's comp)"  bin_pt1=15  sr_2=amp  arith_type2=Unsigned  bin_pt2=0  sr_3=3  arith_type3=Unsigned  bin_pt3=0  sr_4=4  arith_type4=Unsigned  bin_pt4=0  dbl_ovrd=off  block_type=bitbasher
  Bus Creator : BusCreator  Inputs=3
  Counter : xbsIndex_r4/Counter  cnt_type=Free Running  cnt_to=Inf  operation=Up  start_count=0  cnt_by_val=1  arith_type=Unsigned  n_bits=3  bin_pt=0  load_pin=off  rst=on  en=on  explicit_period=off  period=1  use_behavioral_HDL=off  implementation=Fabric  dbl_ovrd=off  block_type=counter
  DDS Compiler 6.0 1 : xbsIndex_r4/DDS Compiler 6.0   partspresent=Phase_Generator_only  dds_clock_rate=100  channels=8  mode_of_operation=Standard  modulus=9  parameter_entry=System_Parameters  spurious_free_dynamic_range=45  frequency_resolution=0.4  noise_shaping=None  phase_width=24  output_width=3  output_selection=Sine_and_Cosine  negative_sine=off  negative_cosine=off  amplitude_mode=Full_Range  memory_type=Auto  optimization_goal=Auto  dsp48_use=Minimal  resync=off  latency_configuration=Auto  latency=1  has_phase_out=on  has_aclken=off  has_aresetn=on  explicit_period=off  period=1  data_has_tlast=Not_Required  has_tready=off  s_phase_has_tuser=User_Field  m_data_has_tuser=Not_Required  m_phase_has_tuser=User_Field  s_phase_tuser_width=7  output_form=Twos_Complement  s_config_sync_mode=On_Vector  phase_increment=Streaming  output_frequency1=0  output_frequency2=0  output_frequency3=0  output_frequency4=0  output_frequency5=0  output_frequency6=0  output_frequency7=0  output_frequency8=0  output_frequency9=0  output_frequency10=0  output_frequency11=0  output_frequency12=0  output_frequency13=0  output_frequency14=0  output_frequency15=0  output_frequency16=0  pinc1='0'  pinc2='0'  pinc3='0'  pinc4='0'  pinc5='0'  pinc6='0'  pinc7='0'  pinc8='0'  pinc9='0'  pinc10='0'  pinc11='0'  pinc12='0'  pinc13='0'  pinc14='0'  pinc15='0'  pinc16='0'  phase_offset=None  phase_offset_angles1=0  phase_offset_angles2=0  phase_offset_angles3=0  phase_offset_angles4=0  phase_offset_angles5=0  phase_offset_angles6=0  phase_offset_angles7=0  phase_offset_angles8=0  phase_offset_angles9=0  phase_offset_angles10=0  phase_offset_angles11=0  phase_offset_angles12=0  phase_offset_angles13=0  phase_offset_angles14=0  phase_offset_angles15=0  phase_offset_angles16=0  poff1='0'  poff2='0'  poff3='0'  poff4='0'  poff5='0'  poff6='0'  poff7='0'  poff8='0'  poff9='0'  poff10='0'  poff11='0'  poff12='0'  poff13='0'  poff14='0'  poff15='0'  poff16='0'  trim_axipin_name=on  simulation_type=hybrid_sim  simulation_model=sysgen:xddsv6_0_cmodel  data_path_portlist={ 's_axis_config_tdata_poff', 's_axis_config_tdata_chan0_poff', 's_axis_config_tdata_pinc', 's_axis_config_tdata_chan0_pinc', 's_axis_phase_tdata_resync', 's_axis_phase_tdata_chan0_resync', 's_axis_phase_tdata_poff', 's_axis_phase_tdata_chan0_poff', 's_axis_phase_tdata_pinc', 's_axis_phase_tdata_chan0_pinc', 's_axis_phase_tdata_phase_in', 'm_axis_data_tdata_sine', 'm_axis_data_tdata_chan0_sine', 'm_axis_data_tdata_cosine', 'm_axis_data_tdata_chan0_cosine', 'm_axis_phase_tdata_phase_out', 'm_axis_phase_tdata_chan0_phase_out'}  por_mode=false  gui_behaviour=Sysgen  ip_name=DDS Compiler  ip_version=6.0  dsptool_ready=true  wrapper_available=true  port_translation_map={ 'aclken' => 'en', 'aresetn' => 'rst' }  ipcore_usecache=true  ipcore_useipmodelcache=true  ipcore_xco_need_fpga_part=true  ipcore_verbose=false  block_type=dds_compiler_v6_0
  DDS Compiler 6.0 2 : xbsIndex_r4/DDS Compiler 6.0   partspresent=SIN_COS_LUT_only  dds_clock_rate=100  channels=1  mode_of_operation=Standard  modulus=9  parameter_entry=System_Parameters  spurious_free_dynamic_range=45  frequency_resolution=0.4  noise_shaping=Taylor_Series_Corrected  phase_width=24  output_width=18  output_selection=Sine_and_Cosine  negative_sine=off  negative_cosine=off  amplitude_mode=Full_Range  memory_type=Auto  optimization_goal=Area  dsp48_use=Minimal  resync=off  latency_configuration=Auto  latency=1  has_phase_out=off  has_aclken=off  has_aresetn=off  explicit_period=off  period=1  data_has_tlast=Not_Required  has_tready=off  s_phase_has_tuser=User_Field  m_data_has_tuser=User_Field  m_phase_has_tuser=Not_Required  s_phase_tuser_width=7  output_form=Twos_Complement  s_config_sync_mode=On_Vector  phase_increment=Streaming  output_frequency1=0  output_frequency2=0  output_frequency3=0  output_frequency4=0  output_frequency5=0  output_frequency6=0  output_frequency7=0  output_frequency8=0  output_frequency9=0  output_frequency10=0  output_frequency11=0  output_frequency12=0  output_frequency13=0  output_frequency14=0  output_frequency15=0  output_frequency16=0  pinc1='0'  pinc2='0'  pinc3='0'  pinc4='0'  pinc5='0'  pinc6='0'  pinc7='0'  pinc8='0'  pinc9='0'  pinc10='0'  pinc11='0'  pinc12='0'  pinc13='0'  pinc14='0'  pinc15='0'  pinc16='0'  phase_offset=Streaming  phase_offset_angles1=0  phase_offset_angles2=0  phase_offset_angles3=0  phase_offset_angles4=0  phase_offset_angles5=0  phase_offset_angles6=0  phase_offset_angles7=0  phase_offset_angles8=0  phase_offset_angles9=0  phase_offset_angles10=0  phase_offset_angles11=0  phase_offset_angles12=0  phase_offset_angles13=0  phase_offset_angles14=0  phase_offset_angles15=0  phase_offset_angles16=0  poff1='0'  poff2='0'  poff3='0'  poff4='0'  poff5='0'  poff6='0'  poff7='0'  poff8='0'  poff9='0'  poff10='0'  poff11='0'  poff12='0'  poff13='0'  poff14='0'  poff15='0'  poff16='0'  trim_axipin_name=on  simulation_type=hybrid_sim  simulation_model=sysgen:xddsv6_0_cmodel  data_path_portlist={ 's_axis_config_tdata_poff', 's_axis_config_tdata_chan0_poff', 's_axis_config_tdata_pinc', 's_axis_config_tdata_chan0_pinc', 's_axis_phase_tdata_resync', 's_axis_phase_tdata_chan0_resync', 's_axis_phase_tdata_poff', 's_axis_phase_tdata_chan0_poff', 's_axis_phase_tdata_pinc', 's_axis_phase_tdata_chan0_pinc', 's_axis_phase_tdata_phase_in', 'm_axis_data_tdata_sine', 'm_axis_data_tdata_chan0_sine', 'm_axis_data_tdata_cosine', 'm_axis_data_tdata_chan0_cosine', 'm_axis_phase_tdata_phase_out', 'm_axis_phase_tdata_chan0_phase_out'}  por_mode=false  gui_behaviour=Sysgen  ip_name=DDS Compiler  ip_version=6.0  dsptool_ready=true  wrapper_available=true  port_translation_map={ 'aclken' => 'en', 'aresetn' => 'rst' }  ipcore_usecache=true  ipcore_useipmodelcache=true  ipcore_xco_need_fpga_part=true  ipcore_verbose=false  block_type=dds_compiler_v6_0
  Inverter : xbsIndex_r4/Inverter  en=off  latency=1  dbl_ovrd=off  block_type=inv
  Register{,1..2,6..11} (9 alike) : xbsIndex_r4/Register  init=0  rst=off  en=off  dbl_ovrd=off  block_type=register
  Register3 : xbsIndex_r4/Register  init=0  rst=off  en=on  dbl_ovrd=off  block_type=register
  Register4 : xbsIndex_r4/Register  init=0  rst=off  en=on  dbl_ovrd=off  block_type=register
  Register5 : xbsIndex_r4/Register  init=0  rst=off  en=on  dbl_ovrd=off  block_type=register
  Terminator1 : Terminator
  Terminator2 : Terminator
  tuser : xbsIndex_r4/Constant  const=0  gui_display_data_type=Boolean  arith_type=Boolean  n_bits=1  bin_pt=0  preci_type=Single  exp_width=8  frac_width=24  explicit_period=off  period=1  equ=P=C  opselect=C  inp2=PCIN>>17  opr=+  inp1=P  carry=CIN  dbl_ovrd=off  block_type=constant
  valid1 : InportShadow
  valid_o : Outport
  Q : Outport  Port=2
  I : Outport  Port=3
  amp_o : Outport  Port=4
  ch_o : Outport  Port=5
  phaseBus : Outport  Port=6
  wires:
  Register10/1 -> BitBasher3/2
  Counter/1 -> Register11/1
  Register11/1 -> Register10/1
  rst/1 -> Inverter/1, Counter/1
  valid/1 -> Counter/2
  Register9/1 -> Register6/1
  Register8/1 -> Register1/1
  Register7/1 -> Register/1
  Inverter/1 -> DDS Compiler 6.0 1/5
  BitBasher5/1 -> Bus Creator/2  "phase"
  Bus Creator/1 -> phaseBus/1
  Register1/1 -> BitBasher2/1
  BitBasher4/1 -> ch_o/1
  Register5/1 -> BitBasher4/1  "INDX"
  BitBasher2/2 -> BitBasher3/1
  freqWord/1 -> Register8/1
  Register2/1 -> valid_o/1  "valid"
  Register3/1 -> Q/1  "Q"
  Register4/1 -> I/1  "I"
  BitBasher/1 -> Register7/1
  ch/1 -> BitBasher/1
  DDS Compiler 6.0 2/2 -> Register3/1  "Q"
  DDS Compiler 6.0 2/1 -> Register5/2, Register4/2, Register3/2, Register2/1  "valid"
  valid1/1 -> Register9/1
  DDS Compiler 6.0 2/3 -> Register4/1  "I"
  DDS Compiler 6.0 2/4 -> Register5/1  "INDX"
  BitBasher4/2 -> amp_o/1
  BitBasher1/1 -> Bus Creator/3  "ch"
  DDS Compiler 6.0 1/1 -> Bus Creator/1, DDS Compiler 6.0 2/1  "valid"
  BitBasher2/1 -> DDS Compiler 6.0 1/2
  BitBasher3/1 -> DDS Compiler 6.0 1/4
  Register6/1 -> DDS Compiler 6.0 1/1  "valid"
  DDS Compiler 6.0 1/2 -> DDS Compiler 6.0 2/2, BitBasher5/1  "phase"
  DDS Compiler 6.0 1/3 -> DDS Compiler 6.0 2/3, BitBasher1/1  "tyser"
  tuser/1 -> DDS Compiler 6.0 1/3
  DDS Compiler 6.0 1/4 -> Terminator1/1
  DDS Compiler 6.0 1/5 -> Terminator2/1

== system CryoDetHcd/DspCore/DSP/channel_processor/channel_processor_x4/128_channel_processor1/DDS Mixer taylor series corrected/mixer ==
  note: depth 16 should be enough
      |   8 here
      |   ~3-4 in DDS block
  note: match latency for phaseBus
  note: Need complex? Swap IQ
  note: can this be modulo 8?
  In1 : Inport
  In2 : Inport  Port=2
  phaseBus : Inport  Port=3
  BitBasher2 : xbsIndex_r4/BitBasher  bitexpr=out={Q, I}  display_expr=off  sr_1=out  arith_type1=Unsigned  bin_pt1=0  sr_2=2  arith_type2=Unsigned  bin_pt2=0  sr_3=3  arith_type3=Unsigned  bin_pt3=0  sr_4=4  arith_type4=Unsigned  bin_pt4=0  dbl_ovrd=off  block_type=bitbasher
  BitBasher3 : xbsIndex_r4/BitBasher  bitexpr=|  display_expr=off  sr_1=Q  arith_type1="Signed  (2's comp)"  bin_pt1=15  sr_2=I  arith_type2="Signed  (2's comp)"  bin_pt2=15  sr_3=I  arith_type3=Unsigned  bin_pt3=0  sr_4=4  arith_type4=Unsigned  bin_pt4=0  dbl_ovrd=off  block_type=bitbasher
      | Q = {in[31:16]}
      | I = {in[15:0]}
  Bus Creator : BusCreator  Inputs=3
  Bus Creator1 : BusCreator  Inputs=4
  Bus Selector1 : BusSelector  OutputSignals=valid,Q,I,ch
  Bus Selector2 : BusSelector  OutputSignals=valid,Q,I
  Bus Selector3 : BusSelector  OutputSignals=valid,phase,ch
  "Complex Multiplier 6.0 " : xbsIndex_r4/Complex Multiplier 6.0   hasatlast=off  hasatuser=on  atuserwidth=3  hasbtlast=off  hasbtuser=off  btuserwidth=1  multtype=Use_Mults  optimizegoal=Resources  flowcontrol=NonBlocking  outputwidth=19  roundmode=Truncate  hasctrltlast=off  hasctrltuser=off  ctrltuserwidth=1  outtlastbehv=Null  latencyconfig=Manual  minimumlatency=6  aclken=off  aresetn=off  trim_axipin_name=on  simulation_type=hybrid_sim  simulation_model=sysgen:cmpy_v6_0  data_path_portlist={ 's_axis_a_tdata_real', 's_axis_a_tdata_imag', 's_axis_b_tdata_real', 's_axis_b_tdata_imag', 's_axis_ctrl_tdata_rounding_bit', 'm_axis_dout_tdata_real', 'm_axis_dout_tdata_imag' }  aportwidth=63  bportwidth=63  ip_name=Complex Multiplier  ip_version=6.0  dsptool_ready=true  ipcore_usecache=true  ipcore_useipmodelcache=true  ipcore_verbose=false  ipcore_latency_parameter='minimumlatency'  wrapper_available=true  port_translation_map={ 'aclken' => 'en', 'aresetn' => 'rst'}  block_type=cmpy_v6_0
  Convert : xbsIndex_r4/Convert  gui_display_data_type=Fixed-point  arith_type="Signed  (2's comp)"  n_bits=18  bin_pt=16  float_type=Single  exp_bits=8  fraction_bits=24  quantization=Truncate  overflow=Wrap  en=off  latency=0  pipeline=off  dbl_ovrd=off  block_type=convert
  Convert1 : xbsIndex_r4/Convert  gui_display_data_type=Fixed-point  arith_type="Signed  (2's comp)"  n_bits=18  bin_pt=16  float_type=Single  exp_bits=8  fraction_bits=24  quantization=Truncate  overflow=Wrap  en=off  latency=0  pipeline=off  dbl_ovrd=off  block_type=convert
  Delay : xbsIndex_r4/Delay  rst=off  infoeditControl=Selection of Reset will increase slice count due to use of real FFs and instead of SRLs  en=off  latency=12  reg_retiming=off  dbl_ovrd=off  block_type=delay
  Delay{1..4,8..11} (8 alike) : xbsIndex_r4/Delay  rst=off  infoeditControl=Selection of Reset will increase slice count due to use of real FFs and instead of SRLs  en=off  latency=1  reg_retiming=on  dbl_ovrd=off  block_type=delay
  Delay12 : xbsIndex_r4/Delay  rst=off  infoeditControl=Selection of Reset will increase slice count due to use of real FFs and instead of SRLs  en=off  latency=16  reg_retiming=off  dbl_ovrd=off  block_type=delay
  Delay5 : xbsIndex_r4/Delay  rst=off  infoeditControl=Selection of Reset will increase slice count due to use of real FFs and instead of SRLs  en=off  latency=12  reg_retiming=off  dbl_ovrd=off  block_type=delay
  Delay6 : xbsIndex_r4/Delay  rst=off  infoeditControl=Selection of Reset will increase slice count due to use of real FFs and instead of SRLs  en=off  latency=16  reg_retiming=off  dbl_ovrd=off  block_type=delay
  Delay7 : xbsIndex_r4/Delay  rst=off  infoeditControl=Selection of Reset will increase slice count due to use of real FFs and instead of SRLs  en=off  latency=16  reg_retiming=off  dbl_ovrd=off  block_type=delay
  downmix : Outport
  phaseBus_o : Outport  Port=2
  wires:
  Delay12/1 -> Bus Creator/3  "ch"
  BitBasher2/1 -> Delay5/1
  BitBasher3/2 -> "Complex Multiplier 6.0 "/6
  Delay5/1 -> BitBasher3/1
  Bus Selector2/1 -> Delay/1  "<valid>"
  Bus Selector2/3 -> BitBasher2/2  "<I>"
  Bus Selector2/2 -> BitBasher2/1  "<Q>"
  Delay/1 -> "Complex Multiplier 6.0 "/5
  Delay2/1 -> "Complex Multiplier 6.0 "/1
  Bus Selector1/1 -> Delay2/1  "<valid>"
  In1/1 -> Bus Selector1/1
  Bus Selector1/2 -> Delay4/1  "<Q>"
  Delay4/1 -> "Complex Multiplier 6.0 "/2
  Bus Selector1/3 -> Delay3/1  "<I>"
  "Complex Multiplier 6.0 "/1 -> Delay8/1  "valid"
  "Complex Multiplier 6.0 "/4 -> Delay11/1  "INDX"
  Delay3/1 -> "Complex Multiplier 6.0 "/3
  "Complex Multiplier 6.0 "/2 -> Convert/1  "Q"
  Delay1/1 -> "Complex Multiplier 6.0 "/4
  BitBasher3/1 -> "Complex Multiplier 6.0 "/7
  "Complex Multiplier 6.0 "/3 -> Convert1/1  "I"
  In2/1 -> Bus Selector2/1
  Bus Selector1/4 -> Delay1/1  "<ch>"
  Convert/1 -> Delay9/1  "Q"
  Convert1/1 -> Delay10/1  "I"
  phaseBus/1 -> Bus Selector3/1
  Bus Selector3/1 -> Delay6/1  "<valid>"
  Bus Selector3/2 -> Delay7/1  "<phase>"
  Bus Selector3/3 -> Delay12/1  "<ch>"
  Delay7/1 -> Bus Creator/2  "phase"
  Delay6/1 -> Bus Creator/1  "valid"
  Bus Creator/1 -> phaseBus_o/1
  Delay10/1 -> Bus Creator1/3  "I"
  Delay11/1 -> Bus Creator1/4  "ch"
  Delay8/1 -> Bus Creator1/1  "valid"
  Delay9/1 -> Bus Creator1/2  "Q"
  Bus Creator1/1 -> downmix/1
